simulink model "simulated_with_compensator"  (R2024b)
settings: Solver=VariableStepAuto  StartTime=0.0  StopTime=10.0  RelTol=1e-3
settings Model: Creator=donadi  LastModifiedBy=donadi

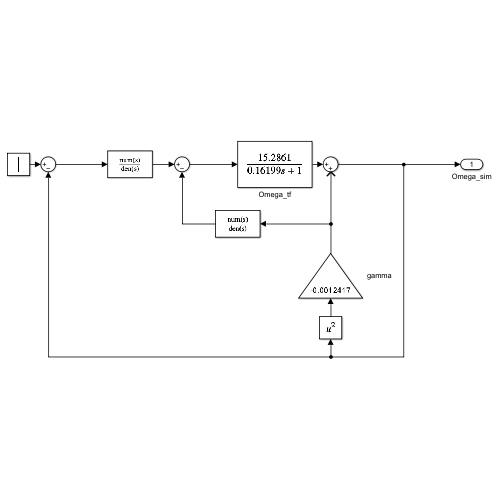
[thumbnail: Simulink's stored preview of the top-level diagram]
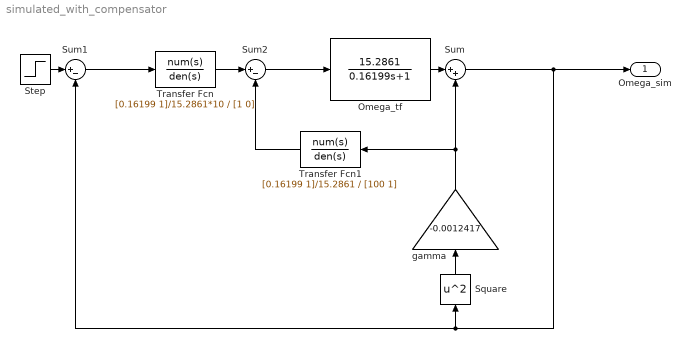
== system simulated_with_compensator ==
  Omega_tf : TransferFcn  Numerator=15.2861  Denominator=[0.16199 1]
  Square : Math  Operator=square
  Step : Step  After=4000  SampleTime=0
  Sum : Sum  Inputs=|++
  Sum1 : Sum  Inputs=|+-
  Sum2 : Sum  Inputs=|+-
  Transfer Fcn : TransferFcn  Numerator=[0.16199 1]/15.2861*10  Denominator=[1 0]
  Transfer Fcn1 : TransferFcn  Numerator=[0.16199 1]/15.2861  Denominator=[100 1]
  gamma : Gain  Gain=-0.0012417
  Omega_sim : Outport
  wires:
  Square/1 -> gamma/1
  gamma/1 -> Transfer Fcn1/1, Sum/2
  Sum/1 -> Sum1/2, Square/1, Omega_sim/1
  Omega_tf/1 -> Sum/1
  Transfer Fcn/1 -> Sum2/1
  Step/1 -> Sum1/1
  Sum2/1 -> Omega_tf/1
  Sum1/1 -> Transfer Fcn/1
  Transfer Fcn1/1 -> Sum2/2
